simulink model "AAI_good"  (R2020a)
settings: Solver=FixedStepAuto  StartTime=0.0  StopTime=10.0  FixedStep=1e-3  RelTol=1e-3  EnableMultiTasking=on
undefined symbols (not defined in the file): D0, D10, D11, D13, D2, D4, D5, D6, D8, PTA0, PTA2, PTB23, PTB9, PTC16, PTC2, PTD0, PTD1, PTD2
libraries: frdmk64flib x9
settings Model: ExtModeTrigDuration=5  Creator=hinda  LastModifiedBy=hinda
settings OptimizationCC: EnhancedBackFolding=on  PassReuseOutputArgsAs=Individual arguments  ZeroExternalMemoryAtStartup=off  ZeroInternalMemoryAtStartup=off  MaxStackSize=64  OptimizeBlockOrder=speed  DifferentSizesBufferReuse=on  OptimizationCustomize=off  EfficientTunableParamExpr=on
settings DebuggingCC: ParameterTunabilityLossMsg=error
settings HardwareCC: ProdBitPerPointer=32  ProdBitPerSizeT=32  ProdBitPerPtrDiffT=32  ProdLargestAtomicInteger=Long  ProdLargestAtomicFloat=Double  ProdWordSize=32  ProdHWDeviceType=ARM Compatible->ARM Cortex
settings SFSimCC: MATLABDynamicMemAlloc=off
settings RTWCC: SystemTargetFile=ert.tlc  HardwareBoard=NXP FRDM-K64F  TemplateMakefile=ert_default_tmf  Toolchain=GNU Tools for ARM Embedded Processors
settings CodeAppCC: ForceParamTrailComments=on  IgnoreCustomStorageClasses=off  OperatorAnnotations=on  SimulinkDataObjDesc=on  SFDataObjDesc=on  InsertBlockDesc=on

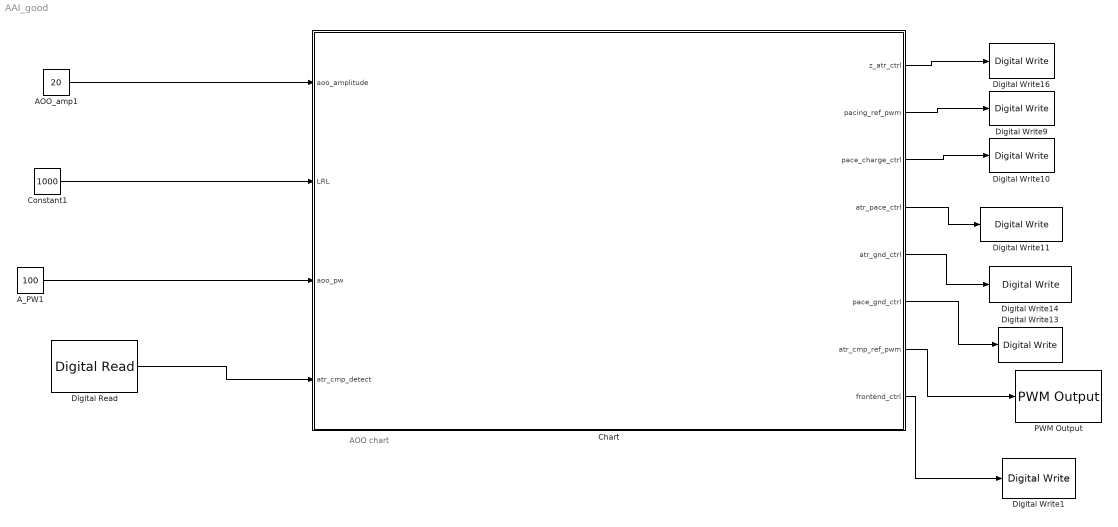
== system AAI_good ==
  note: AOO chart
  AOO_amp1 : Constant  Value=20
  A_PW1 : Constant  Value=100
  Chart : Stateflow chart  TreatAsAtomicUnit=on
  Constant1 : Constant  Value=1000
  Digital Read : frdmk64flib/Digital Read  Whichpin=PTC16 (D0)  SampleTime=-1
  Digital Write1 : frdmk64flib/Digital Write  Whichpin=PTD1 (D13)
  Digital Write10 : frdmk64flib/Digital Write  Whichpin=PTB9 (D2)
  Digital Write11 : frdmk64flib/Digital Write  Whichpin=PTA0 (D8)
  Digital Write13 : frdmk64flib/Digital Write  Whichpin=PTD0 (D10)
  Digital Write14 : frdmk64flib/Digital Write  Whichpin=PTD2 (D11)
  Digital Write16 : frdmk64flib/Digital Write  Whichpin=PTB23 (D4)
  Digital Write9 : frdmk64flib/Digital Write  Whichpin=PTA2 (D5)
  PWM Output : frdmk64flib/PWM Output  Whichpin=PTC2 (D6)  InitialFrequency=2000  InitialDutyCycle=0
  wires:
  Constant1/1 -> Chart/2(LRL)
  AOO_amp1/1 -> Chart/1(aoo_amplitude)
  Chart/4(atr_pace_ctrl) -> Digital Write11/1
  Chart/3(pace_charge_ctrl) -> Digital Write10/1
  Chart/6(pace_gnd_ctrl) -> Digital Write13/1
  A_PW1/1 -> Chart/3(aoo_pw)
  Chart/5(atr_gnd_ctrl) -> Digital Write14/1
  Chart/1(z_atr_ctrl) -> Digital Write16/1
  Chart/2(pacing_ref_pwm) -> Digital Write9/1
  Chart/7(atr_cmp_ref_pwm) -> PWM Output/1
  Digital Read/1 -> Chart/4(atr_cmp_detect)
  Chart/8(frontend_ctrl) -> Digital Write1/1

== stateflow chart AAI_good/Chart ==
  state charging
    entry:
    %charging C22
    %discharging C21
    atr_pace_ctrl = 0; %do not want c22 to discharge
    pacing_ref_pwm = aoo_amplitude; %send in signal
    pace_charge_ctrl = 1;
    pace_gnd_ctrl = 0; %discharges C21
    atr_gnd_ctrl = 1; %1 when discharging through atrium
    %average threshold amplitude is 80
    z_atr_ctrl = 0; %connects impedance circuit to atrium ring electrode output is at z_signal pin
    %sensing
    frontend_ctrl = 1;
    atr_cmp_ref_pwm = 80; %send in threshold signal, if heart is less then we will send signal
  state pacing
    entry:
    %charging C21
    %discharging C22
    atr_gnd_ctrl = 0;
    atr_pace_ctrl = 1;
    z_atr_ctrl = 0;
    pace_charge_ctrl = 0;
    pace_gnd_ctrl = 1;
    pacing_ref_pwm = aoo_amplitude;
    frontend_ctrl = 0;
  (junction 61) -> charging [order 1] : [atr_cmp_detect == 1]
  (default) -> charging
  charging -> (junction 61)
  (junction 61) -> pacing [order 2] : after(LRL-aoo_pw, msec)[atr_cmp_detect==0]
  pacing -> charging : [after(aoo_pw, msec)]
  data: aoo_amplitude input; LRL input; aoo_pw input; z_atr_ctrl output; pacing_ref_pwm output; pace_charge_ctrl output; atr_pace_ctrl output; atr_gnd_ctrl output; pace_gnd_ctrl output; atr_cmp_ref_pwm output; atr_cmp_detect input; frontend_ctrl output
